simulink model "gm_Model"  (R2025a)
settings: Solver=FixedStepDiscrete  StartTime=0.0  StopTime=80000/fs_in  RelTol=1e-3
undefined symbols (not defined in the file or in its folder): a, b, b_fixp, beta_retanh, c, cos_omega, cos_omega_fixp, diag_count, exp_omega, exp_omega_fixp, fixp_chebacc_frac, fixp_chebacc_ws, fixp_dsp_ws, fixp_eig_frac, fixp_eig_ws, fs_in, group_size, hann_table_fixp, image_seed, image_seed_fixp, J_ROM, k, K_ROM, lap_diags, lap_main, lap_main_fi, lap_offsets, lap_offsets_fi, lap_rest, lap_rest_fi, laplacian_diags_main, laplacian_diags_offsets, laplacian_diags_rest, lut_norm_x, lut_norm_y, magnitude, n_ch, n_layer, n_px, n_px_fi, nf, norm_gain_floor, power_iters, power_norm_scaling_factor_fixp, tau, tau_fixp, theta, theta_fixp
libraries: simulink x59, hdlsllib x36, hdlstreaminglib x4, hdlmdlgenlib x1, matrix_library x1, dspvision x1
(part 1 of 8)
settings Model: SimulationMode=accelerator  Creator=bramh  LastModifiedBy=bramh
settings SolverCC: AlgebraicLoopSolver=TrustRegion
settings DataIOCC: LimitDataPoints=on  SaveOutput=off  SaveTime=off
settings OptimizationCC: BlockReduction=off  ConditionallyExecuteInputs=off  DefaultParameterBehavior=Inlined  InheritOutputTypeSmallerThanSingle=on  LifeSpan=inf  SimCompilerOptimization=on
settings DebuggingCC: ReadBeforeWriteMsg=DisableAll  WriteAfterWriteMsg=DisableAll  WriteAfterReadMsg=DisableAll  AlgebraicLoopMsg=error  InheritedTsInSrcMsg=none  MultiTaskDSMMsg=none  SingleTaskRateTransMsg=error  UnconnectedInputMsg=warning  UnconnectedOutputMsg=warning  UnconnectedLineMsg=warning  AllowSymbolicDim=off  StrictBusMsg=ErrorOnBusTreatedAsVector  SFUnexpectedBacktrackingDiag=warning  SFNoUnconditionalDefaultTransitionDiag=warning  SFExecutionAtInitializationDiag=none  ArithmeticOperatorsInVariantConditions=warning
settings HardwareCC: ProdBitPerPointer=32.0  ProdBitPerSizeT=32.0  ProdBitPerPtrDiffT=32.0  ProdLargestAtomicFloat=None  ProdIntDivRoundTo=Undefined  ProdEndianess=Unspecified  ProdWordSize=32.0  ProdHWDeviceType=ASIC/FPGA->ASIC/FPGA  ProdEqTarget=off
settings ModelReferenceCC: EnableRefExpFcnMdlSchedulingChecks=on
settings SFSimCC: SimUseLocalCustomCode=off  CustomCodeUndefinedFunction=UseInterfaceOnly  SimHardwareAcceleration=native
settings RTWCC: RTWUseLocalCustomCode=off  GPUComputeCapability=3.5
settings CodeAppCC: StateflowObjectComments=on
settings GRTTargetCC: TargetLangStandard=C89/C90 (ANSI)
settings ConfigComp: CovScope=ReferencedModels  CovMetricSettings=dw  CovSaveCumulativeToWorkspaceVar=on  CovSaveSingleToWorkspaceVar=on  CovExternalEMLEnable=off  CovSFcnEnable=off

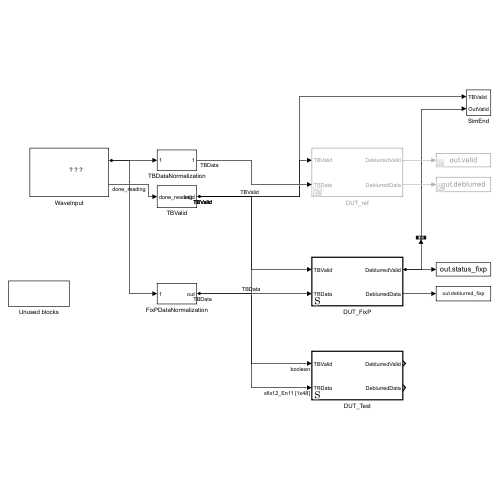
[thumbnail: Simulink's stored preview of the top-level diagram]
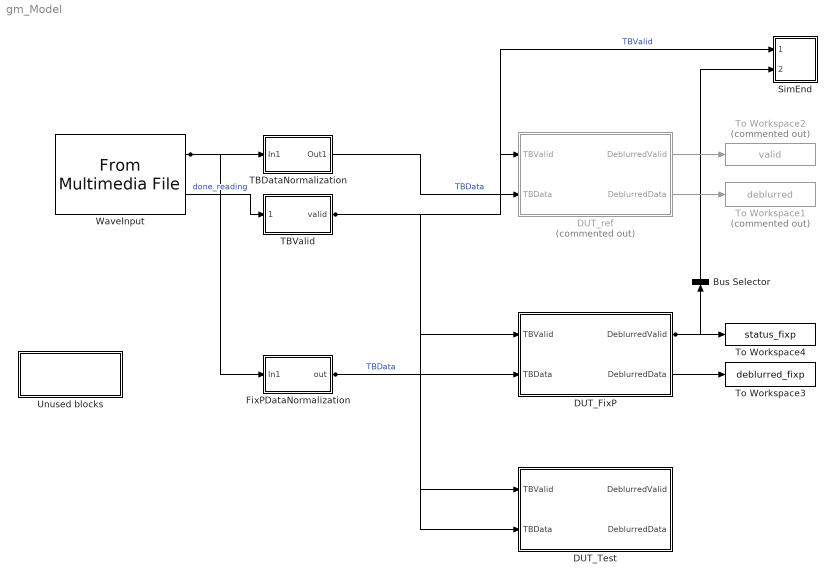
== system gm_Model ==
  Bus Selector : BusSelector  OutputSignals=valid
  DUT_FixP : Subsystem  TreatAsAtomicUnit=on
  DUT_Test : Subsystem  TreatAsAtomicUnit=on
  DUT_ref : Subsystem  Commented=on
  FixPDataNormalization : Subsystem
  SimEnd : Subsystem
  TBDataNormalization : Subsystem
  TBValid : Subsystem
  To Workspace1 : ToWorkspace  Commented=on  VariableName=deblurred  SaveFormat=Timeseries  SampleTime=-1
  To Workspace2 : ToWorkspace  Commented=on  VariableName=valid  SaveFormat=Timeseries  SampleTime=-1
  To Workspace3 : ToWorkspace  VariableName=deblurred_fixp  SaveFormat=Timeseries  SampleTime=-1
  To Workspace4 : ToWorkspace  VariableName=status_fixp  SaveFormat=Timeseries  SampleTime=-1
  Unused blocks : Subsystem
  WaveInput : dspvision/From Multimedia File  inputFilename=wav_file  readRange=[1 Inf]  loop=on  numPlays=1  outputStreams=Audio only  videoDataType=single  audioDataType=int16  inheritSampleTime=on  userDefinedSampleTime=1/30  noAudioOutput=off  isIntensityVideo=off  fourcc=RGB  colorVideoFormat=One multidimensional signal  outputEOF=on  dataOrg=Column-major  audioFrameSize=1  computeAudioFrameSize=off  outSamplingMode=Sample based
      settings: LibrarySourceBlock=dspsrcs4/From Multimedia File
  wires:
  Bus Selector/1 -> SimEnd/2(OutValid)
  DUT_FixP/2(DeblurredData) -> To Workspace3/1
  DUT_FixP/1(DeblurredValid) -> Bus Selector/1, To Workspace4/1
  FixPDataNormalization/1(out) -> DUT_FixP/2(TBData), DUT_Test/2(TBData)  "TBData"
  DUT_ref/2(DeblurredData) -> To Workspace1/1
  TBDataNormalization/1(Out1) -> DUT_ref/2(TBData)  "TBData"
  DUT_ref/1(DeblurredValid) -> To Workspace2/1
  WaveInput/1 -> TBDataNormalization/1(In1), FixPDataNormalization/1(In1)
  WaveInput/2 -> TBValid/1(done_reading)  "done_reading"
  TBValid/1(valid) -> DUT_ref/1(TBValid), SimEnd/1(TBValid), DUT_FixP/1(TBValid), DUT_Test/1(TBValid)  "TBValid"

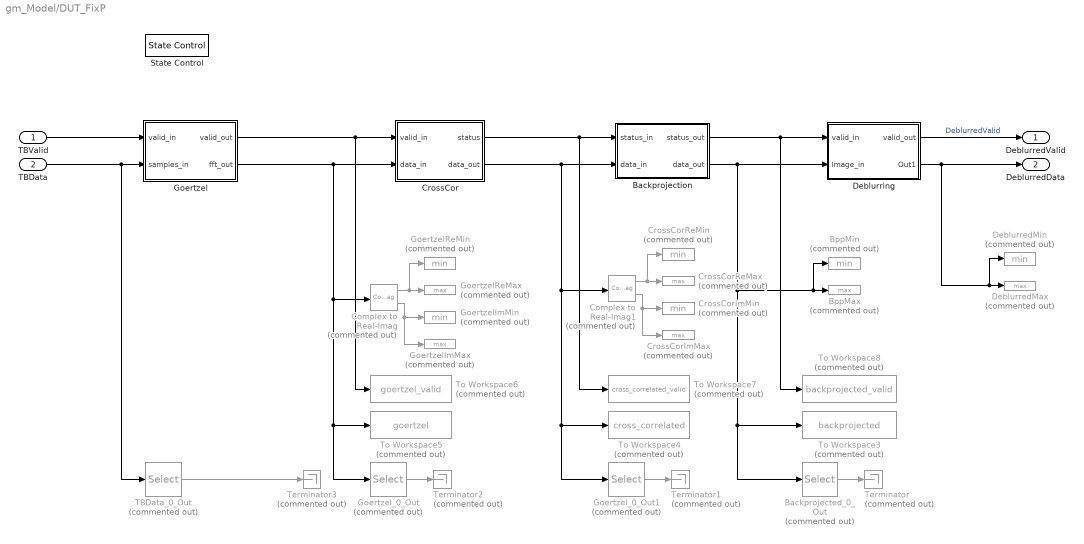
== system gm_Model/DUT_FixP ==
  TBValid : Inport
  TBData : Inport  Port=2
  Backprojected_0_Out : Selector  Commented=on  InputPortWidth=n_px  IndexOptions=Index vector (dialog)  Indices=1  OutputSizes=1
  Backprojection : Subsystem
  BppMax : MinMax  Commented=on  Function=max
  BppMin : MinMax  Commented=on
  Complex to Real-Imag : ComplexToRealImag  Commented=on
  Complex to Real-Imag1 : ComplexToRealImag  Commented=on
  CrossCor : Subsystem
  CrossCorImMax : MinMax  Commented=on  Function=max
  CrossCorImMin : MinMax  Commented=on
  CrossCorReMax : MinMax  Commented=on  Function=max
  CrossCorReMin : MinMax  Commented=on
  DeblurredMax : MinMax  Commented=on  Function=max
  DeblurredMin : MinMax  Commented=on
  Deblurring : Subsystem
  Goertzel : Subsystem
  GoertzelImMax : MinMax  Commented=on  Function=max
  GoertzelImMin : MinMax  Commented=on
  GoertzelReMax : MinMax  Commented=on  Function=max
  GoertzelReMin : MinMax  Commented=on
  Goertzel_0_Out : Selector  Commented=on  InputPortWidth=48  IndexOptions=Index vector (dialog)  Indices=1  OutputSizes=1
  Goertzel_0_Out1 : Selector  Commented=on  NumberOfDimensions=2  InputPortWidth=48  IndexOptions=Index vector (dialog),Index vector (dialog)  Indices=1,1  OutputSizes=1,1
  State Control : StateControl  StateControl=Synchronous
  TBData_0_Out : Selector  Commented=on  InputPortWidth=48  IndexOptions=Index vector (dialog)  Indices=1  OutputSizes=1
  Terminator{,1..3} (4 alike) : Terminator  Commented=on
  To Workspace3 : ToWorkspace  Commented=on  VariableName=backprojected  SaveFormat=Timeseries  SampleTime=-1
  To Workspace4 : ToWorkspace  Commented=on  VariableName=cross_correlated  SaveFormat=Timeseries  SampleTime=-1
  To Workspace5 : ToWorkspace  Commented=on  VariableName=goertzel  SaveFormat=Timeseries  SampleTime=-1
  To Workspace6 : ToWorkspace  Commented=on  VariableName=goertzel_valid  SaveFormat=Timeseries  SampleTime=-1
  To Workspace7 : ToWorkspace  Commented=on  VariableName=cross_correlated_valid  SaveFormat=Timeseries  SampleTime=-1
  To Workspace8 : ToWorkspace  Commented=on  VariableName=backprojected_valid  SaveFormat=Timeseries  SampleTime=-1
  DeblurredValid : Outport
  DeblurredData : Outport  Port=2
  wires:
  Backprojection/2(data_out) -> Backprojected_0_Out/1, To Workspace3/1, BppMax/1, BppMin/1, Deblurring/2(Image_in)
  CrossCor/2(data_out) -> Backprojection/2(data_in), To Workspace4/1, Goertzel_0_Out1/1, Complex to Real-Imag1/1
  Goertzel/2(fft_out) -> CrossCor/2(data_in), Goertzel_0_Out/1, To Workspace5/1, Complex to Real-Imag/1
  Goertzel/1(valid_out) -> CrossCor/1(valid_in), To Workspace6/1
  Deblurring/2(Out1) -> DeblurredData/1, DeblurredMax/1, DeblurredMin/1
  Complex to Real-Imag1/1 -> CrossCorReMax/1, CrossCorReMin/1
  Complex to Real-Imag1/2 -> CrossCorImMin/1, CrossCorImMax/1
  Complex to Real-Imag/2 -> GoertzelImMin/1, GoertzelImMax/1
  Complex to Real-Imag/1 -> GoertzelReMax/1, GoertzelReMin/1
  Goertzel_0_Out/1 -> Terminator2/1
  Backprojected_0_Out/1 -> Terminator/1
  TBData_0_Out/1 -> Terminator3/1
  Deblurring/1(valid_out) -> DeblurredValid/1  "DeblurredValid"
  Goertzel_0_Out1/1 -> Terminator1/1
  Backprojection/1(status_out) -> Deblurring/1(valid_in), To Workspace8/1
  TBData/1 -> Goertzel/2(samples_in), TBData_0_Out/1
  TBValid/1 -> Goertzel/1(valid_in)
  CrossCor/1(status) -> Backprojection/1(status_in), To Workspace7/1

== system gm_Model/DUT_Test ==
  TBValid : Inport  OutDataTypeStr=boolean  PortDimensions=1  SampleTime=6.25e-05
  TBData : Inport  Port=2  OutDataTypeStr=fixdt(1, 12, 11)  PortDimensions=[1 48]  SampleTime=6.25e-05
  CrossCor : Subsystem
  Goertzel : Subsystem
  StateControl : StateControl  StateControl=Synchronous
  bus_selector : BusSelector  OutputSignals=valid
  ctr_0_199 : hdlsllib/Sources/HDL Counter  CountType=Count limited  CountInit=double(0)  CountStep=double(1)  CountMax=double(199)  CountFromType=Initial value  CountFrom=double(0)  CountResetPort=off  CountLoadPort=off  CountEnbPort=off  CountDirPort=off  CountHitOutputPort=off  CountDataType=Unsigned  CountWordLen=8  CountFracLen=0  CountSampTime=3.125e-07
  ctr_0_359999 : hdlsllib/Sources/HDL Counter  CountType=Count limited  CountInit=double(0)  CountStep=double(1)  CountMax=double(359999)  CountFromType=Initial value  CountFrom=double(0)  CountResetPort=off  CountLoadPort=off  CountEnbPort=off  CountDirPort=off  CountHitOutputPort=off  CountDataType=Unsigned  CountWordLen=19  CountFracLen=0  CountSampTime=3.125e-07
  ctr_0_39999 : hdlsllib/Sources/HDL Counter  CountType=Count limited  CountInit=double(0)  CountStep=double(1)  CountMax=double(39999)  CountFromType=Initial value  CountFrom=double(0)  CountResetPort=off  CountLoadPort=off  CountEnbPort=off  CountDirPort=off  CountHitOutputPort=off  CountDataType=Unsigned  CountWordLen=16  CountFracLen=0  CountSampTime=3.125e-07
  t : RateTransition  InitialCondition=double(0)  OutPortSampleTimeOpt=Multiple of input port sample time  OutPortSampleTimeMultiple=360000
  DeblurredValid : Outport  SampleTime=0.1125
  DeblurredData : Outport  Port=2  SampleTime=0.1125
  wires:
  TBValid/1 -> Goertzel/1(valid_in)
  CrossCor/1(status) -> bus_selector/1
  Goertzel/2(fft_out) -> CrossCor/2(data_in)
  ctr_0_199/1 -> Goertzel/3(sch_ctr_199)
  TBData/1 -> Goertzel/2(samples_in)
  ctr_0_39999/1 -> CrossCor/4(sch_ctr_39999)
  Goertzel/1(valid_out) -> CrossCor/1(valid_in)
  ctr_0_359999/1 -> CrossCor/3(sch_ctr_359999)
  CrossCor/2(data_out) -> DeblurredData/1
  bus_selector/1 -> t/1  "<valid>"
  t/1 -> DeblurredValid/1

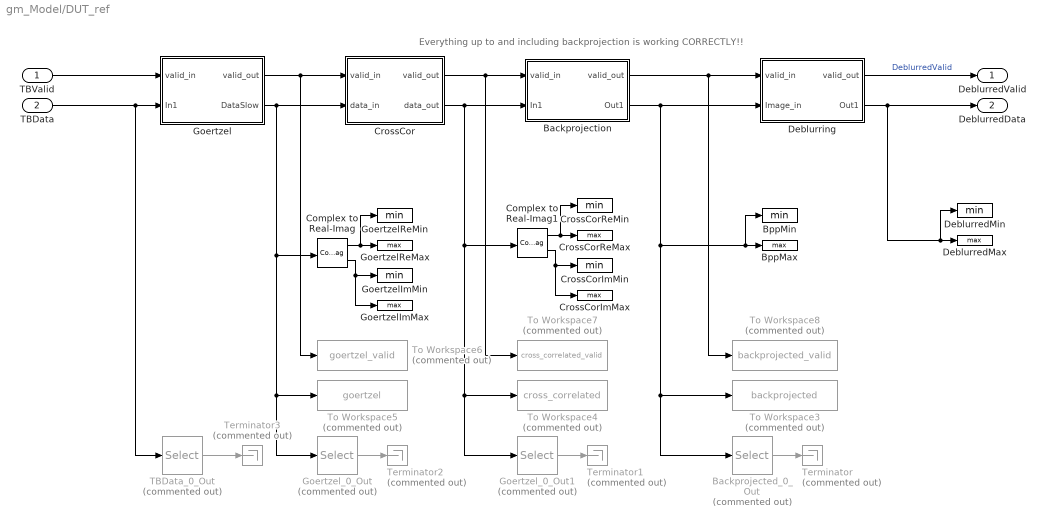
== system gm_Model/DUT_ref ==
  note: Everything up to and including backprojection is working CORRECTLY!!
  TBValid : Inport
  TBData : Inport  Port=2
  Backprojected_0_Out : Selector  Commented=on  InputPortWidth=n_px  IndexOptions=Index vector (dialog)  Indices=1  OutputSizes=1
  Backprojection : Subsystem
  BppMax : MinMax  Function=max
  BppMin : MinMax
  Complex to Real-Imag : ComplexToRealImag
  Complex to Real-Imag1 : ComplexToRealImag
  CrossCor : Subsystem
  CrossCorImMax : MinMax  Function=max
  CrossCorImMin : MinMax
  CrossCorReMax : MinMax  Function=max
  CrossCorReMin : MinMax
  DeblurredMax : MinMax  Function=max
  DeblurredMin : MinMax
  Deblurring : Subsystem
  Goertzel : Subsystem
  GoertzelImMax : MinMax  Function=max
  GoertzelImMin : MinMax
  GoertzelReMax : MinMax  Function=max
  GoertzelReMin : MinMax
  Goertzel_0_Out : Selector  Commented=on  InputPortWidth=48  IndexOptions=Index vector (dialog)  Indices=1  OutputSizes=1
  Goertzel_0_Out1 : Selector  Commented=on  NumberOfDimensions=2  InputPortWidth=48  IndexOptions=Index vector (dialog),Index vector (dialog)  Indices=1,1  OutputSizes=1,1
  TBData_0_Out : Selector  Commented=on  InputPortWidth=48  IndexOptions=Index vector (dialog)  Indices=1  OutputSizes=1
  Terminator{,1..3} (4 alike) : Terminator  Commented=on
  To Workspace3 : ToWorkspace  Commented=on  VariableName=backprojected  SaveFormat=Timeseries  SampleTime=-1
  To Workspace4 : ToWorkspace  Commented=on  VariableName=cross_correlated  SaveFormat=Timeseries  SampleTime=-1
  To Workspace5 : ToWorkspace  Commented=on  VariableName=goertzel  SaveFormat=Timeseries  SampleTime=-1
  To Workspace6 : ToWorkspace  Commented=on  VariableName=goertzel_valid  SaveFormat=Timeseries  SampleTime=-1
  To Workspace7 : ToWorkspace  Commented=on  VariableName=cross_correlated_valid  SaveFormat=Timeseries  SampleTime=-1
  To Workspace8 : ToWorkspace  Commented=on  VariableName=backprojected_valid  SaveFormat=Timeseries  SampleTime=-1
  DeblurredValid : Outport
  DeblurredData : Outport  Port=2
  wires:
  Deblurring/2(Out1) -> DeblurredData/1, DeblurredMax/1, DeblurredMin/1
  Backprojection/2(Out1) -> Deblurring/2(Image_in), Backprojected_0_Out/1, To Workspace3/1, BppMax/1, BppMin/1
  Complex to Real-Imag1/1 -> CrossCorReMax/1, CrossCorReMin/1
  Complex to Real-Imag1/2 -> CrossCorImMin/1, CrossCorImMax/1
  Complex to Real-Imag/2 -> GoertzelImMin/1, GoertzelImMax/1
  Complex to Real-Imag/1 -> GoertzelReMax/1, GoertzelReMin/1
  Goertzel/2(DataSlow) -> CrossCor/2(data_in), Goertzel_0_Out/1, To Workspace5/1, Complex to Real-Imag/1
  Goertzel_0_Out/1 -> Terminator2/1
  CrossCor/2(data_out) -> Backprojection/2(In1), To Workspace4/1, Goertzel_0_Out1/1, Complex to Real-Imag1/1
  Backprojected_0_Out/1 -> Terminator/1
  TBData_0_Out/1 -> Terminator3/1
  Deblurring/1(valid_out) -> DeblurredValid/1  "DeblurredValid"
  Goertzel_0_Out1/1 -> Terminator1/1
  Goertzel/1(valid_out) -> CrossCor/1(valid_in), To Workspace6/1
  Backprojection/1(valid_out) -> Deblurring/1(valid_in), To Workspace8/1
  TBData/1 -> Goertzel/2(In1), TBData_0_Out/1
  TBValid/1 -> Goertzel/1(valid_in)
  CrossCor/1(valid_out) -> Backprojection/1(valid_in), To Workspace7/1

== system gm_Model/FixPDataNormalization ==
  In1 : Inport
  Cast2 : DataTypeConversion  OutDataTypeStr=fixdt(1,fixp_input_ws,fixp_input_ws-1)  ConvertRealWorld=Stored Integer (SI)  RndMeth=Floor
  out : Outport
  wires:
  In1/1 -> Cast2/1
  Cast2/1 -> out/1

== system gm_Model/SimEnd ==
  TBValid : Inport
  OutValid : Inport  Port=2
  NOT2 : Logic  Operator=NOT  IconShape=distinctive  AllPortsSameDT=off  OutDataTypeStr=boolean
  OR1 : Logic  Operator=OR  IconShape=distinctive  AllPortsSameDT=off  OutDataTypeStr=boolean
  Rate Transition : RateTransition  OutPortSampleTimeOpt=Inherit
  Stop Simulation : Stop
  wires:
  OutValid/1 -> Rate Transition/1
  TBValid/1 -> OR1/1
  Rate Transition/1 -> OR1/2
  OR1/1 -> NOT2/1
  NOT2/1 -> Stop Simulation/1

== system gm_Model/TBDataNormalization ==
  In1 : Inport
  Cast To Double : DataTypeConversion  OutDataTypeStr=double  SaturateOnIntegerOverflow=off  RndMeth=Floor
  Constant : Constant  Value=2048
  Divide : Product  Inputs=*/
  Selector : Selector  InputPortWidth=48  IndexOptions=Index vector (dialog)  Indices=1  OutputSizes=1
  Out1 : Outport
  wires:
  Divide/1 -> Out1/1, Selector/1
  In1/1 -> Cast To Double/1
  Cast To Double/1 -> Divide/1
  Constant/1 -> Divide/2

== system gm_Model/TBValid ==
  note: Infinite high latch
  done_reading : Inport
  Delay : Delay  DelayLength=1
  NOT1 : Logic  Operator=NOT  IconShape=distinctive  AllPortsSameDT=off  OutDataTypeStr=boolean
  OR : Logic  Operator=OR  IconShape=distinctive  AllPortsSameDT=off  OutDataTypeStr=boolean
  valid : Outport
  wires:
  NOT1/1 -> valid/1
  done_reading/1 -> OR/1
  OR/1 -> Delay/1, NOT1/1
  Delay/1 -> OR/2

== system gm_Model/Unused blocks ==
  BackprojOpt : Subsystem  Commented=on  TreatAsAtomicUnit=on  mask{b=b, tau=tau}
  Cast : DataTypeConversion  Commented=on  SaturateOnIntegerOverflow=off  RndMeth=Floor
  Cast To Double : DataTypeConversion  Commented=on  OutDataTypeStr=double  SaturateOnIntegerOverflow=off  RndMeth=Floor
  For Each Subsystem : Subsystem  Commented=on  TreatAsAtomicUnit=on
  LapMultiply : MATLAB Function  Commented=on  TreatAsAtomicUnit=on
  wires:
  Cast To Double/1 -> LapMultiply/1(image_in)
  LapMultiply/1(out) -> Cast/1

== system gm_Model/DUT_FixP/Backprojection ==
  status_in : Inport
  data_in : Inport  Port=2
  BackprojNaive : Subsystem  TreatAsAtomicUnit=on  mask{b=b_fixp, tau=tau_fixp}
  Delay : Delay
  status_out : Outport
  data_out : Outport  Port=2
  wires:
  Delay/1 -> status_out/1
  data_in/1 -> BackprojNaive/1(In1)
  status_in/1 -> Delay/1
  BackprojNaive/1(Out1) -> data_out/1

== system gm_Model/DUT_FixP/CrossCor ==
  valid_in : Inport
  data_in : Inport  Port=2
  Bus Creator : BusCreator  Commented=on  Inputs=3
  Bus Creator2 : BusCreator  Inputs=3
  Compare To Constant : simulink/Logic and Bit Operations/Compare To Constant  Commented=on  relop=<  const=norm_gain_floor  OutDataTypeStr=boolean
  Compare To Constant2 : simulink/Logic and Bit Operations/Compare To Constant  relop=<  const=norm_gain_floor  OutDataTypeStr=boolean
  Correlation : Subsystem
  Delay : Delay  DelayLength=1
  Grouping : Subsystem
  NormalizationEig : Subsystem  Commented=on
  NormalizationPower : Subsystem
  status : Outport
  data_out : Outport  Port=2
  wires:
  NormalizationPower/2(data_out) -> data_out/1
  Bus Creator2/1 -> status/1
  Compare To Constant2/1 -> Bus Creator2/2  "norm_floor_hit"
  NormalizationPower/3(norm_out) -> Compare To Constant2/1, Bus Creator2/3  "norm"
  NormalizationPower/1(valid_out) -> Bus Creator2/1  "valid"
  Delay/1 -> Grouping/1(valid_in)
  NormalizationEig/3(Eig_value) -> Compare To Constant/1, Bus Creator/3  "eig"
  Grouping/2(out) -> NormalizationEig/2(out), NormalizationPower/2(out)
  Correlation/1(in) -> Grouping/2(in)
  Compare To Constant/1 -> Bus Creator/2  "norm_gain_floor"
  NormalizationEig/1(valid_out) -> Bus Creator/1  "eig_valid"
  Grouping/1(valid) -> NormalizationEig/1(valid_in), NormalizationPower/1(valid_in)  "valid"
  valid_in/1 -> Delay/1
  data_in/1 -> Correlation/1(In1)

== system gm_Model/DUT_FixP/Deblurring ==
  valid_in : Inport
  Image_in : Inport  Port=2
  Chebyshev : Subsystem
  Delay : Delay  DelayLength=1
  Delay2 : Delay  DelayLength=1
  ImageSeed : Constant  Value=image_seed_fixp  SampleTime=-1
  LayerCounter : hdlsllib/Sources/HDL Counter  CountType=Count limited  CountInit=0  CountStep=1  CountMax=n_layer-1  CountFromType=Initial value  CountFrom=0  CountResetPort=off  CountLoadPort=off  CountEnbPort=off  CountDirPort=off  CountHitOutputPort=off  CountDataType=Unsigned  CountWordLen=ceil(log2(n_layer))  CountFracLen=0  CountSampTime=-1
  MakeSigned : DataTypeConversion  OutDataTypeStr=fixdt(1,fixp_dbl_ws,fixp_dbl_frac)  SaturateOnIntegerOverflow=off  RndMeth=Floor
  Rate Transition : RateTransition  OutPortSampleTimeOpt=Multiple of input port sample time  OutPortSampleTimeMultiple=1/n_layer  OutPortSampleTime=n_layer
  Rate Transition1 : RateTransition  OutPortSampleTimeOpt=Multiple of input port sample time  OutPortSampleTimeMultiple=1/n_layer  OutPortSampleTime=n_layer
  Rate Transition2 : RateTransition  OutPortSampleTimeOpt=Multiple of input port sample time  OutPortSampleTimeMultiple=n_layer  OutPortSampleTime=n_layer
  Rate Transition3 : RateTransition  OutPortSampleTimeOpt=Multiple of input port sample time  OutPortSampleTimeMultiple=n_layer  OutPortSampleTime=n_layer
  Sum : Sum  Inputs=++|  OutDataTypeStr=fixdt(0,fixp_dbl_ws,fixp_dbl_frac)  AccumDataTypeStr=fixdt(1,fixp_dbl_ws,fixp_dbl_frac)  SaturateOnIntegerOverflow=on
  Switch : Switch  Criteria=u2 > Threshold  SaturateOnIntegerOverflow=off  InputSameDT=off
  valid_out : Outport
  Out1 : Outport  Port=2
  wires:
  Switch/1 -> Chebyshev/1(Image_in)
  MakeSigned/1 -> Delay2/1
  Rate Transition3/1 -> Out1/1
  Chebyshev/1(Out1) -> Sum/2
  Rate Transition/1 -> MakeSigned/1
  Sum/1 -> Switch/1, Rate Transition3/1
  Delay2/1 -> Sum/1
  Delay/1 -> Rate Transition2/1
  ImageSeed/1 -> Switch/3
  Rate Transition2/1 -> valid_out/1  "ValidOutSlow"
  Rate Transition1/1 -> Delay/1  "ValidInFast"
  valid_in/1 -> Rate Transition1/1  "ValidInSlow"
  Image_in/1 -> Rate Transition/1
  LayerCounter/1 -> Switch/2

== system gm_Model/DUT_FixP/Goertzel ==
  valid_in : Inport
  samples_in : Inport  Port=2
  DataValidDownsampler : Subsystem
  EnabledGoertzel : Subsystem
  valid_out : Outport
  fft_out : Outport  Port=2
  wires:
  DataValidDownsampler/2(DataSlow) -> fft_out/1
  DataValidDownsampler/1(ValidSlow) -> valid_out/1
  EnabledGoertzel/1(valid_out) -> DataValidDownsampler/1(ValidFast)
  EnabledGoertzel/2(Out1) -> DataValidDownsampler/2(DataFast)
  valid_in/1 -> EnabledGoertzel/Enable
  samples_in/1 -> EnabledGoertzel/1(samples_in)
